simulink model "P4"  (R2017a)
settings: Solver=ode45  StartTime=0.0  StopTime=120  RelTol=1e-3
values from neighbouring files (symbols this model uses):
  Kd = Kp*(0.5*L)    [Untitled.m]
  Ki = Kp/(2*L)    [Untitled.m]
  Kp = 1.2*(Tau/L)    [Untitled.m]
libraries: simulink x6
settings Model: Creator=Propietario  LastModifiedBy=Propietario

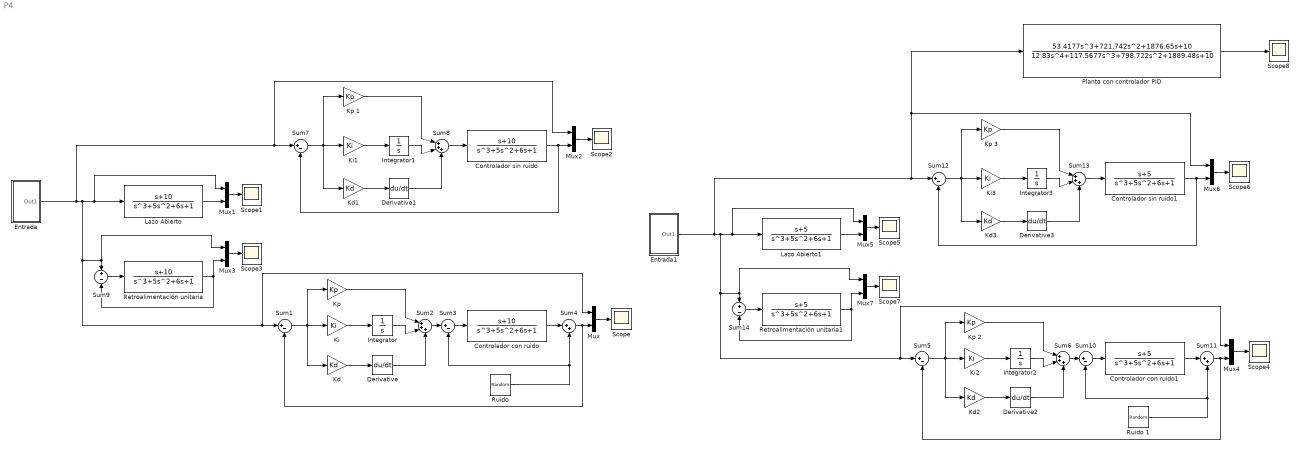
== system P4 ==
  Controlador con ruido : TransferFcn  Numerator=[1 10]  Denominator=[1 5 6 1]
  Controlador con ruido1 : TransferFcn  Numerator=[1 5]  Denominator=[1 5 6 1]
  Controlador sin ruido : TransferFcn  Numerator=[1 10]  Denominator=[1 5 6 1]
  Controlador sin ruido1 : TransferFcn  Numerator=[1 5]  Denominator=[1 5 6 1]
  Derivative{,1..3} (4 alike) : Derivative
  Entrada : Subsystem
  Entrada1 : Subsystem
  Integrator{,1..3} (4 alike) : Integrator
  Kd{,1..3} (4 alike) : Gain  Gain=Kd
  Ki{,1..3} (4 alike) : Gain  Gain=Ki
  Kp {,1..3} (4 alike) : Gain  Gain=Kp
  Lazo Abierto : TransferFcn  Numerator=[1 10]  Denominator=[1 5 6 1]
  Lazo Abierto1 : TransferFcn  Numerator=[1 5]  Denominator=[1 5 6 1]
  Mux{,1..7} (8 alike) : Mux  Inputs=2
  Planta con controlador PID : TransferFcn  Numerator=[0,53.4177,721.742,1876.65,10]  Denominator=[12.83,117.5677,798.722,1889.48,10]
  Retroalimentación unitaria : TransferFcn  Numerator=[1 10]  Denominator=[1 5 6 1]
  Retroalimentación unitaria1 : TransferFcn  Numerator=[1 5]  Denominator=[1 5 6 1]
  "Ruido " : UniformRandomNumber  Minimum=-0.2  Maximum=0.2  SampleTime=5
  Ruido 1 : UniformRandomNumber  Minimum=-0.2  Maximum=0.2  SampleTime=5
  Scope{,1..8} (9 alike) : Scope
  Sum{1,3,5,7,10,12} (6 alike) : Sum  Inputs=|+-
  Sum11 : Sum  Inputs=|++
  Sum{2,6,8,13} (4 alike) : Sum  Inputs=|+++
  Sum14 : Sum  Inputs=+-
  Sum4 : Sum  Inputs=|++
  Sum9 : Sum  Inputs=+-
  wires:
  Mux/1 -> Scope/1
  Sum1/1 -> Kd/1, "Kp "/1, Ki/1
  Ki/1 -> Integrator/1
  "Kp "/1 -> Sum2/1
  Integrator/1 -> Sum2/2
  Kd/1 -> Derivative/1
  Derivative/1 -> Sum2/3
  Sum2/1 -> Sum3/1
  Sum3/1 -> Controlador con ruido/1
  Sum4/1 -> Sum1/2, Mux/2
  Controlador con ruido/1 -> Sum4/1
  "Ruido "/1 -> Sum3/2, Sum4/2
  Mux1/1 -> Scope1/1
  Mux2/1 -> Scope2/1
  Controlador sin ruido/1 -> Mux2/2, Sum7/2
  Sum8/1 -> Controlador sin ruido/1
  Kd1/1 -> Derivative1/1
  Integrator1/1 -> Sum8/2
  Sum7/1 -> Kd1/1, Kp 1/1, Ki1/1
  Kp 1/1 -> Sum8/1
  Derivative1/1 -> Sum8/3
  Ki1/1 -> Integrator1/1
  Mux3/1 -> Scope3/1
  Retroalimentación unitaria/1 -> Mux3/2, Sum9/2
  Sum9/1 -> Retroalimentación unitaria/1
  Entrada/1(Out1) -> Sum1/1, Mux/1, Mux3/1, Sum9/1, Lazo Abierto/1, Mux1/1, Mux2/1, Sum7/1
  Lazo Abierto/1 -> Mux1/2
  Kp 2/1 -> Sum6/1
  Sum14/1 -> Retroalimentación unitaria1/1
  Mux5/1 -> Scope5/1
  Kd2/1 -> Derivative2/1
  Sum12/1 -> Kd3/1, Kp 3/1, Ki3/1
  Kp 3/1 -> Sum13/1
  Sum13/1 -> Controlador sin ruido1/1
  Derivative3/1 -> Sum13/3
  Integrator3/1 -> Sum13/2
  Ki3/1 -> Integrator3/1
  Retroalimentación unitaria1/1 -> Mux7/2, Sum14/2
  Sum5/1 -> Kd2/1, Kp 2/1, Ki2/1
  Mux4/1 -> Scope4/1
  Kd3/1 -> Derivative3/1
  Sum10/1 -> Controlador con ruido1/1
  Controlador sin ruido1/1 -> Mux6/2, Sum12/2
  Mux6/1 -> Scope6/1
  Derivative2/1 -> Sum6/3
  Ruido 1/1 -> Sum10/2, Sum11/2
  Lazo Abierto1/1 -> Mux5/2
  Controlador con ruido1/1 -> Sum11/1
  Mux7/1 -> Scope7/1
  Ki2/1 -> Integrator2/1
  Sum11/1 -> Sum5/2, Mux4/2
  Sum6/1 -> Sum10/1
  Integrator2/1 -> Sum6/2
  Planta con controlador PID/1 -> Scope8/1
  Entrada1/1(Out1) -> Sum5/1, Mux4/1, Mux7/1, Sum14/1, Lazo Abierto1/1, Mux5/1, Planta con controlador PID/1, Mux6/1, Sum12/1

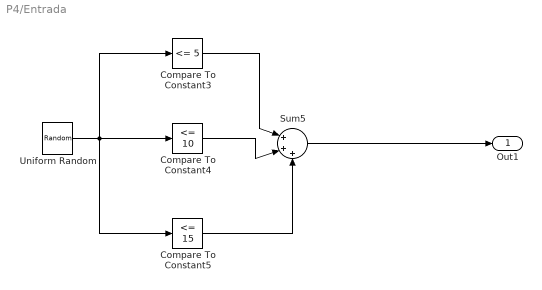
== system P4/Entrada ==
  Compare To Constant3 : simulink/Logic and Bit Operations/Compare To Constant  relop=<=  const=5  OutDataTypeStr=uint8
  Compare To Constant4 : simulink/Logic and Bit Operations/Compare To Constant  relop=<=  const=10  OutDataTypeStr=uint8
  Compare To Constant5 : simulink/Logic and Bit Operations/Compare To Constant  relop=<=  const=15  OutDataTypeStr=uint8
  Sum5 : Sum  Inputs=|+++  OutDataTypeStr=double  LockScale=on
  "Uniform Random " : UniformRandomNumber  Minimum=0  Maximum=20  SampleTime=5
  Out1 : Outport
  wires:
  "Uniform Random "/1 -> Compare To Constant5/1, Compare To Constant3/1, Compare To Constant4/1
  Compare To Constant4/1 -> Sum5/2
  Compare To Constant5/1 -> Sum5/3
  Compare To Constant3/1 -> Sum5/1
  Sum5/1 -> Out1/1

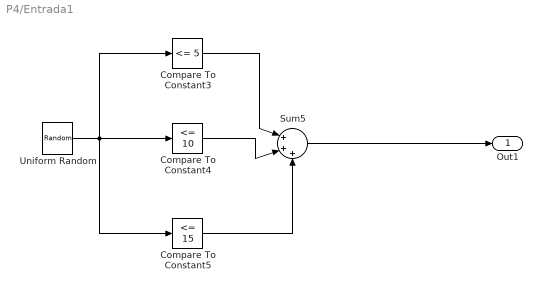
== system P4/Entrada1 ==
  Compare To Constant3 : simulink/Logic and Bit Operations/Compare To Constant  relop=<=  const=5  OutDataTypeStr=uint8
  Compare To Constant4 : simulink/Logic and Bit Operations/Compare To Constant  relop=<=  const=10  OutDataTypeStr=uint8
  Compare To Constant5 : simulink/Logic and Bit Operations/Compare To Constant  relop=<=  const=15  OutDataTypeStr=uint8
  Sum5 : Sum  Inputs=|+++  OutDataTypeStr=double  LockScale=on
  "Uniform Random " : UniformRandomNumber  Minimum=0  Maximum=20  SampleTime=5
  Out1 : Outport
  wires:
  "Uniform Random "/1 -> Compare To Constant5/1, Compare To Constant3/1, Compare To Constant4/1
  Compare To Constant4/1 -> Sum5/2
  Compare To Constant5/1 -> Sum5/3
  Compare To Constant3/1 -> Sum5/1
  Sum5/1 -> Out1/1
